simulink model "ADAC_AEBS_Test_B3_cs"  (Simulink 7.6)
settings: Solver=ode5  SolverMode=SingleTasking  StartTime=0.0  StopTime=inf  FixedStep=1/100  RelTol=1e-3
model workspace (MAT data in the model file):
  mbox_table : struct (value not decoded)
  model_closed = 0
  sim_status = 0
PreLoadFcn:
  | check_NUTS_defined;
  | 
  | assignin('base',['model_closed_' bdroot],false);addpath('../includes_AEBS');
InitFcn:
  | PreScanExperimentInitFcn(bdroot)
StopFcn:
  | PreScanExperimentStopFcn(bdroot)
undefined symbols (not defined in the file): DiscIntNeverNeededParam, x_ini_VRML, y_ini_VRML, z_ini_VRML
libraries: simulink x24, PreScanSimulinkLibrary x12, simulink_extras x7, PreScanUsefulBlocks x5, simulink_need_slupdate x1
(part 1 of 5)
CloseFcn:
  | evalin('base',['clear model_closed_' bdroot]);
settings Model: Creator=PRESCAN  LastModifiedBy=buildbot  BufferReuse=off
settings OptimizationCC: OptimizeBlockIOStorage=off  BufferReuse=off  ExpressionFolding=off  LocalBlockOutputs=off  InitFltsAndDblsToZero=on
settings DebuggingCC: SaveWithParameterizedLinksMsg=none  SignalResolutionControl=TryResolveAllWithWarning  SolverPrmCheckMsg=none  MultiTaskDSMMsg=warning  MultiTaskCondExecSysMsg=none
settings RTWCC: IncludeERTFirstTime=on
settings GRTTargetCC: TargetFcnLib=ansi_tfl_tmw.mat

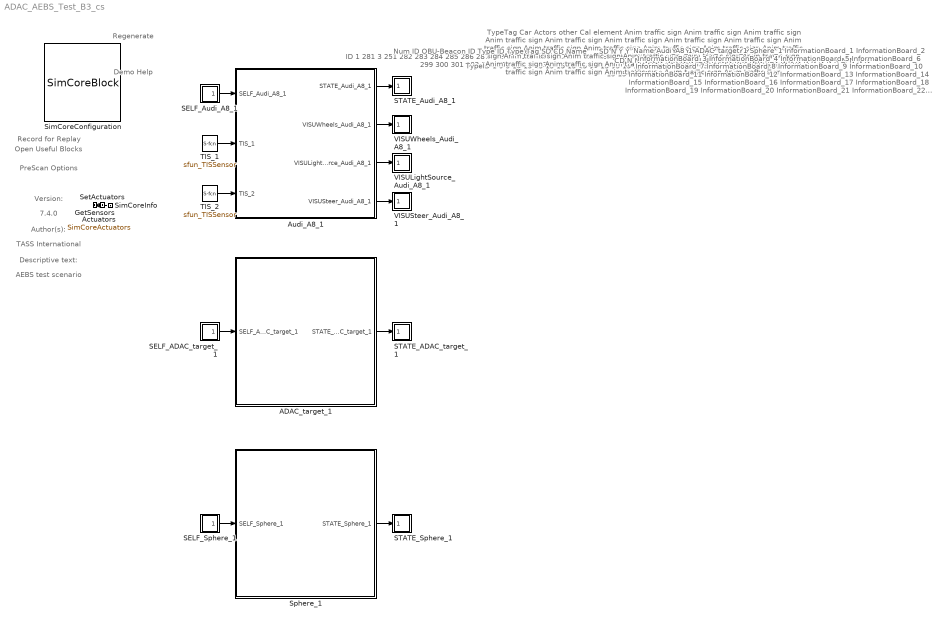
== system ADAC_AEBS_Test_B3_cs ==
  note: Demo Help
  note: Regenerate
  note: Record for Replay
  note: Open Useful Blocks
  note: PreScan Options
  note: Version:
  note: 7.4.0
  note: Author(s):
  note: TASS International
  note: Descriptive text:
  note: AEBS test scenario
  note: ID
      |
      | 1
      | 281
      | 3
      | 251
      | 282
      | 283
      | 284
      | 285
      | 286
      | 287
      | 288
      | 289
      | 290
      | 291
      | 292
      | 293
      | 294
      | 295
      | 296
      | 297
      | 298
      | 299
      | 300
      | 301
      | 302
      | 303
      | 304
      | 305
      | 306
      | 307
      | 308
      | 309
  note: OBU-Beacon ID
  note: TypeID
      |
      | 1
      | 9
      | 5
      | 15
      | 15
      | 15
      | 15
      | 15
      | 15
      | 15
      | 15
      | 15
      | 15
      | 15
      | 15
      | 15
      | 15
      | 15
      | 15
      | 15
      | 15
      | 15
      | 15
      | 15
      | 15
      | 15
      | 15
      | 15
      | 15
      | 15
      | 15
      | 15
  note: TypeTag
      |
      | Car
      | Actors other
      | Cal element
      | Anim traffic sign
      | Anim traffic sign
      | Anim traffic sign
      | Anim traffic sign
      | Anim traffic sign
      | Anim traffic sign
      | Anim traffic sign
      | Anim traffic sign
      | Anim traffic sign
      | Anim traffic sign
      | Anim traffic sign
      | Anim traffic sign
      | Anim traffic sign
      | Anim traffic sign
      | Anim traffic sign
      | Anim traffic sign
      | Anim traffic sign
      | Anim traffic sign
      | Anim traffic sign
      | Anim traffic sign
      | Anim traffic sign
      | Anim traffic sign
      | Anim traffic sign
      | Anim traffic sign
      | Anim traffic sign
      | Anim traffic sign
      | Anim traffic sign
      | Anim traffic sign
      | Anim traffic sign
  note: SD
      |
      | N
      | Y
      | Y
      | Y
      | Y
      | Y
      | Y
      | Y
      | Y
      | Y
      | Y
      | Y
      | Y
      | Y
      | Y
      | Y
      | Y
      | Y
      | Y
      | Y
      | Y
      | Y
      | Y
      | Y
      | Y
      | Y
      | Y
      | Y
      | Y
      | Y
      | Y
      | Y
  note: CD
      |
      | N
      | N
      | N
      | N
      | N
      | N
      | N
      | N
      | N
      | N
      | N
      | N
      | N
      | N
      | N
      | N
      | N
      | N
      | N
      | N
      | N
      | N
      | N
      | N
      | N
      | N
      | N
      | N
      | N
      | N
      | N
      | N
  note: Name
      |
      | Audi_A8_1
      | ADAC_target_1
      | Sphere_1
      | InformationBoard_1
      | InformationBoard_2
      | InformationBoard_3
      | InformationBoard_4
      | InformationBoard_5
      | InformationBoard_6
      | InformationBoard_7
      | InformationBoard_8
      | InformationBoard_9
      | InformationBoard_10
      | InformationBoard_11
      | InformationBoard_12
      | InformationBoard_13
      | InformationBoard_14
      | InformationBoard_15
      | InformationBoard_16
      | InformationBoard_17
      | InformationBoard_18
      | InformationBoard_19
      | InformationBoard_20
      | InformationBoard_21
      | InformationBoard_22
      | InformationBoard_23
      | InformationBoard_24
      | InformationBoard_25
      | InformationBoard_26
      | InformationBoard_27
      | InformationBoard_28
      | InformationBoard_29
  note: Num ID OBU-Beacon ID Type ID Type Tag SD CD Name
  ADAC_target_1 : Subsystem  Tag=WorldObjectSubSystem  InitFcn=UniqueId = '402';
      mask Display: image(imread('ADAC_target.jpg'));color('white');text(0,0,' ID=281\n')
  Actuators : DataStoreMemory  Tag=Actuators  DataStoreName=SimCoreActuators  InitialValue=zeros(273,1)
      settings: DeleteFcn=PreScanBlockDeleteFcn;
  Audi_A8_1 : Subsystem  Tag=WorldObjectSubSystem  InitFcn=UniqueId = '13';
      mask Display: image(imread('Audi_A8.jpg'));color('white');text(0,0,' ID=1\n')
  GetSensors : Subsystem  Tag=GetSensors  Priority=2  mask(PreScan Simulation Core Block){NrOfSensors=24, TimeStep=1/100}
      mask prompts: NrOfSensors "Number of sensor values"; TimeStep "Timestep [s]"
      mask help:
      | Please do not remove this block from the PreScan compilation sheet,
      | as it contains essential configuration parameters for a PreScan simulation.
      settings: DeleteFcn=PreScanBlockDeleteFcn;
  SELF_ADAC_target_1 : Subsystem  Tag=SELF  Priority=3  mask(PreScan Source Block: SELF){PortName=SELF_ADAC_target_1, PortIndex=8, PortWidth=8, TimeStep=1/100}
      mask prompts: PortName "Auto-Assigned: Port Name [-]"; PortIndex "Auto-Assigned: Port Index [-]"; PortWidth "Auto-Assigned: Port Dimensions"; TimeStep "Auto-Assigned: Upload Period [s]"
      mask help:
      | The SELF port shows (state) information of the actor itself. The outputs are position in the experiment's axis system and the GPS coordinates, and the object's absolute velocity and compass heading.
      |
      | For more information, please click Help.
      settings: DeleteFcn=PreScanBlockDeleteFcn;
      mask Help: eval('openHelp(462)')
      mask Display: image(imread('GPS.png'))
  SELF_Audi_A8_1 : Subsystem  Tag=SELF  Priority=3  mask(PreScan Source Block: SELF){PortName=SELF_Audi_A8_1, PortIndex=0, PortWidth=8, TimeStep=1/100}
      mask prompts: PortName "Auto-Assigned: Port Name [-]"; PortIndex "Auto-Assigned: Port Index [-]"; PortWidth "Auto-Assigned: Port Dimensions"; TimeStep "Auto-Assigned: Upload Period [s]"
      mask help:
      | The SELF port shows (state) information of the actor itself. The outputs are position in the experiment's axis system and the GPS coordinates, and the object's absolute velocity and compass heading.
      |
      | For more information, please click Help.
      settings: DeleteFcn=PreScanBlockDeleteFcn;
      mask Help: eval('openHelp(462)')
      mask Display: image(imread('GPS.png'))
  SELF_Sphere_1 : Subsystem  Tag=SELF  Priority=3  mask(PreScan Source Block: SELF){PortName=SELF_Sphere_1, PortIndex=16, PortWidth=8, TimeStep=1/100}
      mask prompts: PortName "Auto-Assigned: Port Name [-]"; PortIndex "Auto-Assigned: Port Index [-]"; PortWidth "Auto-Assigned: Port Dimensions"; TimeStep "Auto-Assigned: Upload Period [s]"
      mask help:
      | The SELF port shows (state) information of the actor itself. The outputs are position in the experiment's axis system and the GPS coordinates, and the object's absolute velocity and compass heading.
      |
      | For more information, please click Help.
      settings: DeleteFcn=PreScanBlockDeleteFcn;
      mask Help: eval('openHelp(462)')
      mask Display: image(imread('GPS.png'))
  STATE_ADAC_target_1 : Subsystem  Tag=State  Priority=0  mask(PreScan Sink Block: State){x0=128, y0=0, z0=0, Roll0=0, Pitch0=0, Yaw0=0, TimeStep=1/100}
      mask prompts: x0 "Ini x-position VEHICLE wrt GLOBAL axis system [m]"; y0 "Ini y-position VEHICLE wrt GLOBAL axis system [m]"; z0 "Ini z-position VEHICLE wrt GLOBAL axis system [m]"; Roll0 "Ini roll-angle BODY wrt VEHICLE axis system [deg]"; Pitch0 "Ini pitch-angle BODY wrt VEHICLE axis system [deg]"; Yaw0 "Ini yaw-angle VEHICLE wrt GLOBAL axis system [deg]"; TimeStep "Time Step [s]"
      mask help:
      | The Actor State contains a vector signal of size (9x1), containing the following signals:
      |
      | -  Position                  (x,y,z)                                     [m]
      | -  Velocity                  (vx,vy,vz)                               [m/s]
      | -  Angles                    (Roll, Pitch, Yaw)                   [rad]
      |
      | The Actor state is defined in the global axis system.
      | The state is superponed on the Initial position defined in the GUI.
      |
      | For more information, please click Help.
      settings: DeleteFcn=PreScanBlockDeleteFcn;
      mask Help: eval('openHelp(222)')
      mask Display: image(imread('State.png'))
  STATE_Audi_A8_1 : Subsystem  Tag=State  Priority=0  mask(PreScan Sink Block: State){x0=-2, y0=0, z0=0.550000011920929, Roll0=0, Pitch0=0, Yaw0=0, TimeStep=1/100}
      mask prompts: x0 "Ini x-position VEHICLE wrt GLOBAL axis system [m]"; y0 "Ini y-position VEHICLE wrt GLOBAL axis system [m]"; z0 "Ini z-position VEHICLE wrt GLOBAL axis system [m]"; Roll0 "Ini roll-angle BODY wrt VEHICLE axis system [deg]"; Pitch0 "Ini pitch-angle BODY wrt VEHICLE axis system [deg]"; Yaw0 "Ini yaw-angle VEHICLE wrt GLOBAL axis system [deg]"; TimeStep "Time Step [s]"
      mask help:
      | The Actor State contains a vector signal of size (9x1), containing the following signals:
      |
      | -  Position                  (x,y,z)                                     [m]
      | -  Velocity                  (vx,vy,vz)                               [m/s]
      | -  Angles                    (Roll, Pitch, Yaw)                   [rad]
      |
      | The Actor state is defined in the global axis system.
      | The state is superponed on the Initial position defined in the GUI.
      |
      | For more information, please click Help.
      settings: DeleteFcn=PreScanBlockDeleteFcn;
      mask Help: eval('openHelp(222)')
      mask Display: image(imread('State.png'))
  STATE_Sphere_1 : Subsystem  Tag=State  Priority=0  mask(PreScan Sink Block: State){x0=-2, y0=0, z0=0.550000011920929, Roll0=0, Pitch0=0, Yaw0=0, TimeStep=1/100}
      mask prompts: x0 "Ini x-position VEHICLE wrt GLOBAL axis system [m]"; y0 "Ini y-position VEHICLE wrt GLOBAL axis system [m]"; z0 "Ini z-position VEHICLE wrt GLOBAL axis system [m]"; Roll0 "Ini roll-angle BODY wrt VEHICLE axis system [deg]"; Pitch0 "Ini pitch-angle BODY wrt VEHICLE axis system [deg]"; Yaw0 "Ini yaw-angle VEHICLE wrt GLOBAL axis system [deg]"; TimeStep "Time Step [s]"
      mask help:
      | The Actor State contains a vector signal of size (9x1), containing the following signals:
      |
      | -  Position                  (x,y,z)                                     [m]
      | -  Velocity                  (vx,vy,vz)                               [m/s]
      | -  Angles                    (Roll, Pitch, Yaw)                   [rad]
      |
      | The Actor state is defined in the global axis system.
      | The state is superponed on the Initial position defined in the GUI.
      |
      | For more information, please click Help.
      settings: DeleteFcn=PreScanBlockDeleteFcn;
      mask Help: eval('openHelp(222)')
      mask Display: image(imread('State.png'))
  SetActuators : Subsystem  Tag=SetActuators  Priority=1  mask(PreScan Simulation Core Block){TimeStep=1/100, NrOfActuators=273}
      mask prompts: TimeStep "Timestep [s]"; NrOfActuators "Number of actuator values"
      mask help:
      | Please do not remove this block from the PreScan compilation sheet,
      | as it contains essential configuration parameters for a PreScan simulation.
      settings: DeleteFcn=PreScanBlockDeleteFcn;
  SimCoreConfiguration : M-S-Function  Tag=SimCoreConfiguration  Description=956F042E7F661D7092DC54456114AB9A9416500EBD947CDBFDED334F67B644E2  FunctionName=SimCoreBlock  Parameters=ExperimentXML PortsXML SimulationCore HostName CheckStart EnableLog RfR EnableGPUAccel ShowComputationTime  mask(PreScan Simulation Core Configurator){SimulationCore=NUTS, HostName=0, CheckStart=0, prescanversion='7.4.0', EnableLog=off, RfR=0, EnableGPUAccel=off, ShowComputationTime=off}
      mask prompts: SimulationCore "Simulation Core"; HostName "Simulation Host"; CheckStart "Show START Dialog"; prescanversion "PreScan Version"; EnableLog "Create TA Log"; RfR "Record for Replay"; EnableGPUAccel "Enable GPU Acceleration"; ShowComputationTime "Show ComputationTime Scope"
      mask help:
      | Please do not remove this block from the PreScan compilation sheet,
      | as it contains essential configuration parameter for a PreScan simulation.
      mask init:
      | model = bdroot;
      | ExperimentXML = [model(1:end-3) '.pex'];
      | PortsXML = [model '_ports.pcd'];
      settings: DeleteFcn=PreScanBlockDeleteFcn;  ModelCloseFcn=assignin('base',['model_closed_' bdroot],true);
      mask Help: eval('openHelp(812)')
      mask Display: image(imread('prescanlogo.ico'))
  SimCoreInfo : Subsystem  Tag=SimCoreInfo
  Sphere_1 : Subsystem  Tag=WorldObjectSubSystem  InitFcn=UniqueId = '409';
      mask Display: image(imread('Sphere.jpg'));color('white');text(0,0,' ID=3\n')
  TIS_1 : S-Function  Priority=3  LoadFcn=load('PrescanScannerSensorData.mat');load('PrescanScannerSensorMessage.mat')  FunctionName=sfun_TISSensor  Parameters=timestepMask maxInputMessages maxOutputMessages sensorID detectableObjects  EnableBusSupport=off  mask{timestepMask=1/25, maxInputMessages=0, maxOutputMessages=32, sensorID=14, detectableObjects=32}
      mask prompts: timestepMask "MATLAB timestep:"; maxInputMessages "Max input messages:"; maxOutputMessages "Max output messages:"; sensorID "Sensor ID:"; detectableObjects "Max detectable objects:"
      mask help: TIS Sensor I/O
      mask Display: image(imread('TIS.png'))
  TIS_2 : S-Function  Priority=3  LoadFcn=load('PrescanScannerSensorData.mat');load('PrescanScannerSensorMessage.mat')  FunctionName=sfun_TISSensor  Parameters=timestepMask maxInputMessages maxOutputMessages sensorID detectableObjects  EnableBusSupport=off  mask{timestepMask=1/25, maxInputMessages=0, maxOutputMessages=32, sensorID=15, detectableObjects=32}
      mask prompts: timestepMask "MATLAB timestep:"; maxInputMessages "Max input messages:"; maxOutputMessages "Max output messages:"; sensorID "Sensor ID:"; detectableObjects "Max detectable objects:"
      mask help: TIS Sensor I/O
      mask Display: image(imread('TIS.png'))
  VISULightSource_Audi_A8_1 : Subsystem  Tag=VisuLightSource  Priority=0
      settings: DeleteFcn=PreScanBlockDeleteFcn;
      mask Type: PreScan Sink Block: VisuLightSource
      mask Description:
      | The VisuLightSource block provides a way to animate Light Sources of the indicator, braking, fog and main lights of a vehicle.
      | 
      | For more information, please click Help.
      mask Help: eval('openHelp(223)')
      mask Display: image(imread('RearLight.png'))
  VISUSteer_Audi_A8_1 : Subsystem  Tag=VisuSteer  Priority=0
      settings: DeleteFcn=PreScanBlockDeleteFcn;
      mask Type: PreScan Sink Block: VisuSteer
      mask Description:
      | The VisuSteer block provides a way to adapt the orientation of the steering column and steering wheel of a vehicle.
      | 
      | For more information, please click Help.
      mask Help: eval('openHelp(223)')
      mask Display: image(imread('steeringwheel.png'))
  VISUWheels_Audi_A8_1 : Subsystem  Tag=VisuWheels  Priority=0
      settings: DeleteFcn=PreScanBlockDeleteFcn;
      mask Type: PreScan Sink Block: VisuWheels
      mask Description:
      | The VisuWheels block provides a way to animate the wheels of a vehicle, with steering, rotation (because of velocity) and z-displacement.
      | 
      | For more information, please click Help.
      mask Help: eval('openHelp(223)')
      mask Display: image(imread('wheel.png'))
  wires:
  Audi_A8_1/1(STATE_Audi_A8_1) -> STATE_Audi_A8_1/1(State)
  SELF_Audi_A8_1/1(U) -> Audi_A8_1/1(SELF_Audi_A8_1)
  TIS_1/1 -> Audi_A8_1/2(TIS_1)
  TIS_2/1 -> Audi_A8_1/3(TIS_2)
  Audi_A8_1/2(VISUWheels_Audi_A8_1) -> VISUWheels_Audi_A8_1/1(Wheels)
  Audi_A8_1/3(VISULightSource_Audi_A8_1) -> VISULightSource_Audi_A8_1/1(Lights)
  Audi_A8_1/4(VISUSteer_Audi_A8_1) -> VISUSteer_Audi_A8_1/1(Steer)
  ADAC_target_1/1(STATE_ADAC_target_1) -> STATE_ADAC_target_1/1(State)
  SELF_ADAC_target_1/1(U) -> ADAC_target_1/1(SELF_ADAC_target_1)
  Sphere_1/1(STATE_Sphere_1) -> STATE_Sphere_1/1(State)
  SELF_Sphere_1/1(U) -> Sphere_1/1(SELF_Sphere_1)
  SetActuators/1(dummy) -> GetSensors/1(dummy)

== system ADAC_AEBS_Test_B3_cs/ADAC_target_1 ==
  SELF_ADAC_target_1 : Inport  Tag=SELFInport
  SELF_Demux : Subsystem  Tag=DemuxSELF
      settings: DeleteFcn=PreScanBlockDeleteFcn;
      mask Type: PreScan Demux Block:
      mask Display:
      | port_label('output',1,'x [m]')
      | port_label('output',2,'y [m]')
      | port_label('output',3,'z [m]','texmode','on')
      | port_label('output',4,'Rotx [deg]','texmode','on')
      | port_label('output',5,'Roty [deg]','texmode','on')
      | port_label('output',6,'Rotz [deg]','texmode','on')
      | port_label('output',7,'GPS lat [deg]','texmode','on')
      | port_label('output',8,'GPS long [deg]','texmode','on')
      | port_label('output',9,'GPS alt [m]','texmode','on')
      | port_label('output',10,'Velocity [m/s]')
      | port_label('output',11,'Heading [deg]')
      | port_label('output',12,'Yaw rate [deg/s]')
  Terminator_{1..12} (12 alike) : Terminator
  Trajectories : Subsystem  Tag=Trajectories
      settings: DeleteFcn=PreScanBlockDeleteFcn;
      mask Type: PreScan Source Block: Trajectories
      mask Description:
      | The Trajectory block contains the trajectories defined in the PreScan Experiment Editor. The output of the trajectory block is the (vehicle) State.
      | 
      | For more information, please click Help.
      mask Help: eval('openHelp(312)')
      mask Display: image(imread('Trajectory.png'));
  STATE_ADAC_target_1 : Outport  Tag=StateOutport
  wires:
  SELF_ADAC_target_1/1 -> SELF_Demux/1(SELF)
  Trajectories/1(State) -> STATE_ADAC_target_1/1
  SELF_Demux/1(x [m]) -> Terminator_1/1
  SELF_Demux/2(y [m]) -> Terminator_2/1
  SELF_Demux/3(z [m]) -> Terminator_3/1
  SELF_Demux/4(rotx [deg]) -> Terminator_4/1
  SELF_Demux/5(roty [deg]) -> Terminator_5/1
  SELF_Demux/6(rotz [deg]) -> Terminator_6/1
  SELF_Demux/7(GPS lat [deg]) -> Terminator_7/1
  SELF_Demux/8(GPS long [deg]) -> Terminator_8/1
  SELF_Demux/9(GPS alt [m]) -> Terminator_9/1
  SELF_Demux/10(velocity [m/s]) -> Terminator_10/1
  SELF_Demux/11(heading [deg]) -> Terminator_11/1
  SELF_Demux/12(yaw rate [deg/s]) -> Terminator_12/1

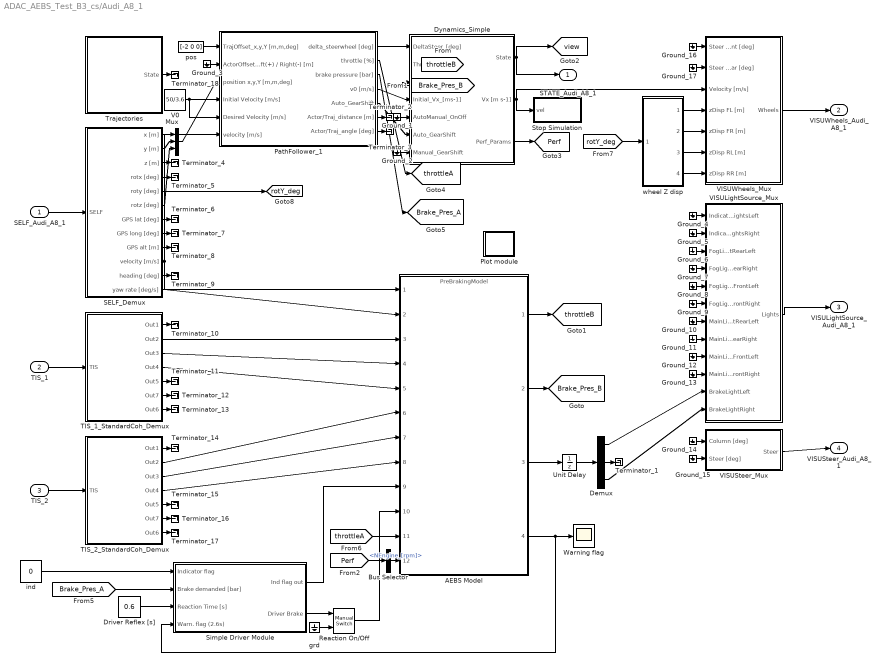
== system ADAC_AEBS_Test_B3_cs/Audi_A8_1 ==
  SELF_Audi_A8_1 : Inport  Tag=SELFInport
  TIS_1 : Inport  Tag=RadarInport  Port=2  OutDataTypeStr=Bus: PRESCAN_SCANNERSENSORMESSAGE
  TIS_2 : Inport  Tag=RadarInport  Port=3  OutDataTypeStr=Bus: PRESCAN_SCANNERSENSORMESSAGE
  AEBS Model : ModelReference  ModelNameDialog=PreBrakingModel  SimulationMode=Normal  ModelReferenceVersion=1.738  CopyOfModelName=PreBrakingModel
  Bus Selector : BusSelector  OutputSignals=NEngine_[rpm]
  Demux : Demux  Outputs=3
  Driver Reflex [s] : Constant  Value=0.6
  Dynamics_Simple : Subsystem  Tag=Simple_Vehicle_Dynamics  mask(PreScan Block: Simple Dynamics){Migrate=on, TimeStep=1/100, ComputationMode=Continuous_Time}
      mask prompts: Migrate "Migrate. During migration this block will be replaced by a newer one."; TimeStep "Auto assigned: Time Step [s]"; ComputationMode "Computation mode:"
      mask help:
      | The Simple Dynamics Model is selected in the GUI to simulate vehicle dynamics behavior.
      |
      | The Simple Dynamics Model is completely open to the user. The parameters of this model can be set in the Simple Dynamics dialog in the GUI.
      |
      | For more information, please click Help.
      mask init:
      | p = SimpleDyn_pars;
      settings: DeleteFcn=PreScanBlockDeleteFcn;
      mask Help: eval('openHelp(220)')
      mask Display:
      | image(imread('SimpleDyn.png'))
      | port_label('input', 1, '{\delta}_S_t_ _e_e_r [deg]','texmode','on')
      | port_label('input', 2, 'Throttle [%]')
      | port_label('input', 3, 'Brake Pres [bar]')
      | port_label('input', 4, 'V_0 [ms-1]','texmode','on')
      | port_label('input', 5, 'Auto=[0]/Manual=[1]')
      | port_label('input', 6, 'Auto_GearShift')
      | port_label('input', 7, 'Manual_GearShift')
      | port_label('output', 1, 'State')
      | port_label('output', 2, 'Vx [ms-1]')
      | port_label('output', 3, 'Perf Params')
  Ground_{1..17} (17 alike) : Ground
  Mux : Mux  Inputs=3
  PathFollower_1 : Subsystem  Tag=pathFollower  mask(PreScan Block: Path Follower){Migrate=on, FileName='Trajectory_2.mat', TunableSteeringGain=1, XShifting_wrt_COG=0}
      mask prompts: Migrate "Migrate. During migration this block will be replaced by a newer one."; FileName "Trajectory Name"; TunableSteeringGain "TunableSteeringGain [-]"; XShifting_wrt_COG "XShifting_wrt_COG [m]"
      mask help:
      | The Path Follower Model is selected in the GUI to simulate driver behavior.
      |
      | For more information, please click Help.
      mask init:
      | load(['trajectories/',eval(FileName)])
      | traject=trajectory';
      | 
      | Traj_x=traject(:,2);
      | Traj_y=traject(:,3);
      | Traj_z=traject(:,4);
      | Traj_vx=traject(:,8);
      | Traj_vy=traject(:,9);
      | Traj_vz=traject(:,10);
      mask Help: eval('openHelp(232)')
  Plot module : Subsystem  StopFcn=|
      | eml.extrinsic('plotyy','AEBS_EGOplot');
      | AEBS_EGOplot;
  Reaction On/Off : simulink/Signal Routing/Manual Switch  SystemSampleTime=-1  sw=0  action=0  varsize=off
  SELF_Demux : Subsystem  Tag=DemuxSELF
      settings: DeleteFcn=PreScanBlockDeleteFcn;
      mask Type: PreScan Demux Block:
      mask Display:
      | port_label('output',1,'x [m]')
      | port_label('output',2,'y [m]')
      | port_label('output',3,'z [m]','texmode','on')
      | port_label('output',4,'Rotx [deg]','texmode','on')
      | port_label('output',5,'Roty [deg]','texmode','on')
      | port_label('output',6,'Rotz [deg]','texmode','on')
      | port_label('output',7,'GPS lat [deg]','texmode','on')
      | port_label('output',8,'GPS long [deg]','texmode','on')
      | port_label('output',9,'GPS alt [m]','texmode','on')
      | port_label('output',10,'Velocity [m/s]')
      | port_label('output',11,'Heading [deg]')
      | port_label('output',12,'Yaw rate [deg/s]')
  Simple Driver Module : Subsystem
  Stop Simulation : Subsystem
  TIS_1_StandardCoh_Demux : Subsystem  TreatAsAtomicUnit=on  mask(PreScan Demux Block: TIS){MAXMESSAGES=32}
      mask prompts: MAXMESSAGES "Number of Objects"
      mask Help: eval('openHelp(441)')
      mask Display:
      | port_label('input',1,'TIS')
      | port_label('output',1,'Beam ID [-]')
      | port_label('output',2,'Range [m]')
      | port_label('output',3,'DopplerVelocity [m/s]')
      | port_label('output',4,'{\theta} [deg]','texmode','on')
      | port_label('output',5,'{\phi} [deg]','texmode','on')
      | port_label('output',6,'Target ID [-]','texmode','on')
      | port_label('output',7,'TIS Data','texmode','on')
  TIS_2_StandardCoh_Demux : Subsystem  TreatAsAtomicUnit=on  mask(PreScan Demux Block: TIS){MAXMESSAGES=32}
      mask prompts: MAXMESSAGES "Number of Objects"
      mask Help: eval('openHelp(441)')
      mask Display:
      | port_label('input',1,'TIS')
      | port_label('output',1,'Beam ID [-]')
      | port_label('output',2,'Range [m]')
      | port_label('output',3,'DopplerVelocity [m/s]')
      | port_label('output',4,'{\theta} [deg]','texmode','on')
      | port_label('output',5,'{\phi} [deg]','texmode','on')
      | port_label('output',6,'Target ID [-]','texmode','on')
      | port_label('output',7,'TIS Data','texmode','on')
  Terminator_{1..18} (18 alike) : Terminator
  Trajectories : Subsystem  Tag=Trajectories
      settings: DeleteFcn=PreScanBlockDeleteFcn;
      mask Type: PreScan Source Block: Trajectories
      mask Description:
      | The Trajectory block contains the trajectories defined in the PreScan Experiment Editor. The output of the trajectory block is the (vehicle) State.
      | 
      | For more information, please click Help.
      mask Help: eval('openHelp(312)')
      mask Display: image(imread('Trajectory.png'));
  Unit Delay : UnitDelay  SampleTime=-1
  V0 : Constant  Value=50/3.6
  VISULightSource_Mux : Subsystem  Tag=MuxLightSource
      settings: DeleteFcn=PreScanBlockDeleteFcn;
      mask Type: PreScan Mux Block:
  VISUSteer_Mux : Subsystem  Tag=MuxSteer
      settings: DeleteFcn=PreScanBlockDeleteFcn;
      mask Type: PreScan Mux Block:
  VISUWheels_Mux : Subsystem  Tag=MuxWheels  mask(PreScan Mux Block:){TimeStep=1/100}
      mask prompts: TimeStep "Auto Assigned: Time Step [s]"
      settings: DeleteFcn=PreScanBlockDeleteFcn;
  Warning flag : Scope
      settings: TimeRange=1.8  YMin=-1  YMax=1
  grd : Ground
  ind : Constant  Value=0
  pos : Constant  Tag=pos  Value=[-2 0 0]
  wheel Z disp : Subsystem  InitFcn=a = 1.17;  mask{a=1.17, b=1.77}
      mask prompts: a "Distance to the front wheel from cars center of gravity [m]"; b "Distance to the back wheel from cars center of gravity [m]"
      mask help: Simple Dynamics parameters
  STATE_Audi_A8_1 : Outport  Tag=StateOutport
  VISUWheels_Audi_A8_1 : Outport  Tag=VisuWheelsOutport  Port=2  SampleTime=1/100
  VISULightSource_Audi_A8_1 : Outport  Tag=VisuLightsOutport  Port=3  SampleTime=1/100
  VISUSteer_Audi_A8_1 : Outport  Tag=VisuSteerOutport  Port=4  SampleTime=1/100
  tag scope: Brake_Pres_A=global, Brake_Pres_B=global, Perf=global, rotY_deg=global, throttleA=global, throttleB=global, view=global
  wires:
  AEBS Model/2 -> [Brake_Pres_B]
  AEBS Model/4 -> Warning flag/1, Simple Driver Module/4(Warn. flag (2.6s))
  AEBS Model/1 -> [throttleB]
  [Brake_Pres_A] -> Simple Driver Module/2(Brake demanded [bar])
  Driver Reflex [s]/1 -> Simple Driver Module/3(Reaction Time [s])
  ind/1 -> Simple Driver Module/1(Indicator flag)
  Simple Driver Module/2(Driver Brake) -> Reaction On/Off/1
  grd/1 -> Reaction On/Off/2
  AEBS Model/3 -> Unit Delay/1
  Simple Driver Module/1(Ind flag out) -> AEBS Model/9
  Reaction On/Off/1 -> AEBS Model/10
  [throttleA] -> AEBS Model/11
  [rotY_deg] -> wheel Z disp/1(rotY [deg])
  Unit Delay/1 -> Demux/1
  [Perf] -> Bus Selector/1
  Bus Selector/1 -> AEBS Model/12  "<NEngine_[rpm]>"
  pos/1 -> PathFollower_1/1(TrajOffset_x,y,Y [m,m,deg])
  SELF_Audi_A8_1/1 -> SELF_Demux/1(SELF)
  VISUWheels_Mux/1(Wheels) -> VISUWheels_Audi_A8_1/1
  VISULightSource_Mux/1(Lights) -> VISULightSource_Audi_A8_1/1
  VISUSteer_Mux/1(Steer) -> VISUSteer_Audi_A8_1/1
  Dynamics_Simple/2(Vx [m s-1]) -> VISUWheels_Mux/3(Velocity [m/s]), Stop Simulation/1(vel)
  PathFollower_1/1(delta_steerwheel [deg]) -> Dynamics_Simple/1(DeltaSteer_[deg])
  PathFollower_1/2(throttle [%]) -> [throttleA]
  PathFollower_1/3(brake pressure [bar]) -> [Brake_Pres_A]
  PathFollower_1/4(v0 [m/s]) -> Dynamics_Simple/4(Initial_Vx_[ms-1])
  PathFollower_1/5(Auto_GearShift) -> Dynamics_Simple/6(Auto_GearShift)
  Dynamics_Simple/1(State) -> STATE_Audi_A8_1/1, [view]
  TIS_2_StandardCoh_Demux/2(Out2) -> AEBS Model/6
  TIS_1_StandardCoh_Demux/2(Out2) -> AEBS Model/3
  TIS_2_StandardCoh_Demux/3(Out3) -> AEBS Model/7
  TIS_1_StandardCoh_Demux/3(Out3) -> AEBS Model/4
  wheel Z disp/4(zDisp RR [m]) -> VISUWheels_Mux/7(zDisp RR [m])
  wheel Z disp/3(zDisp RL [m]) -> VISUWheels_Mux/6(zDisp RL [m])
  wheel Z disp/2(zDisp FR [m]) -> VISUWheels_Mux/5(zDisp FR [m])
  wheel Z disp/1(zDisp FL [m]) -> VISUWheels_Mux/4(zDisp FL [m])
  SELF_Demux/5(roty [deg]) -> [rotY_deg]
  Demux/3 -> VISULightSource_Mux/12(BrakeLightRight)
  Demux/1 -> VISULightSource_Mux/11(BrakeLightLeft)
  V0/1 -> PathFollower_1/4(Initial Velocity [m/s]), PathFollower_1/5(Desired Velocity [m/s])
  Mux/1 -> PathFollower_1/3(position x,y,Y [m,m,deg])
  SELF_Demux/6(rotz [deg]) -> Mux/3
  SELF_Demux/2(y [m]) -> Mux/2
  SELF_Demux/1(x [m]) -> Mux/1
  Dynamics_Simple/3(Perf_Params) -> [Perf]
  [throttleB] -> Dynamics_Simple/2(Throttle)
  [Brake_Pres_B] -> Dynamics_Simple/3(Brake)
  SELF_Demux/10(velocity [m/s]) -> PathFollower_1/6(velocity [m/s]), AEBS Model/1
  SELF_Demux/12(yaw rate [deg/s]) -> AEBS Model/2
  TIS_1_StandardCoh_Demux/4(Out4) -> AEBS Model/5
  TIS_2_StandardCoh_Demux/4(Out4) -> AEBS Model/8
  TIS_1/1 -> TIS_1_StandardCoh_Demux/1(TIS)
  TIS_2/1 -> TIS_2_StandardCoh_Demux/1(TIS)
  Demux/2 -> Terminator_1/1
  Ground_1/1 -> Dynamics_Simple/5(AutoManual_OnOff)
  Ground_2/1 -> Dynamics_Simple/7(Manual_GearShift)
  Ground_3/1 -> PathFollower_1/2(ActorOffset_Left(+) / Right(-) [m])
  PathFollower_1/6(Actor/Traj_distance [m]) -> Terminator_2/1
  PathFollower_1/7(Actor/Traj_angle [deg]) -> Terminator_3/1
  SELF_Demux/3(z [m]) -> Terminator_4/1
  SELF_Demux/4(rotx [deg]) -> Terminator_5/1
  SELF_Demux/7(GPS lat [deg]) -> Terminator_6/1
  SELF_Demux/8(GPS long [deg]) -> Terminator_7/1
  SELF_Demux/9(GPS alt [m]) -> Terminator_8/1
  SELF_Demux/11(heading [deg]) -> Terminator_9/1
  TIS_1_StandardCoh_Demux/1(Out1) -> Terminator_10/1
  TIS_1_StandardCoh_Demux/5(Out5) -> Terminator_11/1
  TIS_1_StandardCoh_Demux/6(Out7) -> Terminator_12/1
  TIS_1_StandardCoh_Demux/7(Out6) -> Terminator_13/1
  TIS_2_StandardCoh_Demux/1(Out1) -> Terminator_14/1
  TIS_2_StandardCoh_Demux/5(Out5) -> Terminator_15/1
  TIS_2_StandardCoh_Demux/6(Out7) -> Terminator_16/1
  TIS_2_StandardCoh_Demux/7(Out6) -> Terminator_17/1
  Trajectories/1(State) -> Terminator_18/1
  Ground_4/1 -> VISULightSource_Mux/1(IndicatorLightsLeft)
  Ground_5/1 -> VISULightSource_Mux/2(IndicatorLightsRight)
  Ground_6/1 -> VISULightSource_Mux/3(FogLightRearLeft)
  Ground_7/1 -> VISULightSource_Mux/4(FogLightRearRight)
  Ground_8/1 -> VISULightSource_Mux/5(FogLightFrontLeft)
  Ground_9/1 -> VISULightSource_Mux/6(FogLightFrontRight)
  Ground_10/1 -> VISULightSource_Mux/7(MainLightRearLeft)
  Ground_11/1 -> VISULightSource_Mux/8(MainLightRearRight)
  Ground_12/1 -> VISULightSource_Mux/9(MainLightFrontLeft)
  Ground_13/1 -> VISULightSource_Mux/10(MainLightFrontRight)
  Ground_14/1 -> VISUSteer_Mux/1(Column [deg])
  Ground_15/1 -> VISUSteer_Mux/2(Steer [deg])
  Ground_16/1 -> VISUWheels_Mux/1(Steer Angle Front [deg])
  Ground_17/1 -> VISUWheels_Mux/2(Steer Angle Rear [deg])

== system ADAC_AEBS_Test_B3_cs/GetSensors ==
  dummy : Inport
  GetSensors : M-S-Function  FunctionName=GetSensorsBlock  Parameters=TimeStep NrOfSensors
  tag scope: SimCoreSensors=global
  wires:
  GetSensors/1 -> [SimCoreSensors]
  dummy/1 -> GetSensors/1

== system ADAC_AEBS_Test_B3_cs/SELF_ADAC_target_1 ==
  Selector : Selector  IndexMode=Zero-based  IndexOptions=Starting index (dialog)  Indices=PortIndex  OutputSizes=PortWidth(1)
  U : Outport
  wires:
  Selector/1 -> U/1
  [SimCoreSensors] -> Selector/1

== system ADAC_AEBS_Test_B3_cs/SELF_Audi_A8_1 ==
  Selector : Selector  IndexMode=Zero-based  IndexOptions=Starting index (dialog)  Indices=PortIndex  OutputSizes=PortWidth(1)
  U : Outport
  wires:
  Selector/1 -> U/1
  [SimCoreSensors] -> Selector/1

== system ADAC_AEBS_Test_B3_cs/SELF_Sphere_1 ==
  Selector : Selector  IndexMode=Zero-based  IndexOptions=Starting index (dialog)  Indices=PortIndex  OutputSizes=PortWidth(1)
  U : Outport
  wires:
  Selector/1 -> U/1
  [SimCoreSensors] -> Selector/1

== system ADAC_AEBS_Test_B3_cs/STATE_ADAC_target_1 ==
  State : Inport  SampleTime=TimeStep
  Acceleration : Subsystem  mask(ToSensorWorld){PortName=Acceleration_ADAC_target_1, PortIndex=249, PortWidth=3, TimeStep=1/100}
      mask prompts: PortName "Port Name [-]"; PortIndex "Index [-]"; PortWidth "Port Dimensions [-]"; TimeStep "Upload Period [s]"
      mask help: Sends signal(s) from Simulink to the Sensor World
      mask Help:
      | Sends signal(s) from Simulink to the Sensor World.
      | 
      | - Port Name [-]: specifies the name of the output terminal of the Simulink block.
      | - Index [-]: specifies the start position in the output vector sent to the Sensor World
      | - Port dimensions [-]: specifies the width (number of scalars) of the output port
      | - Upload period [s]: specifies the upload period (in seconds) of the port.
      mask Display: port_label('input', 1, PortName)
  Demux : Demux  Outputs=5
  Position : Subsystem  mask(ToSensorWorld){PortName=Position_ADAC_target_1, PortIndex=243, PortWidth=3, TimeStep=1/100}
      mask prompts: PortName "Port Name [-]"; PortIndex "Index [-]"; PortWidth "Port Dimensions [-]"; TimeStep "Upload Period [s]"
      mask help: Sends signal(s) from Simulink to the Sensor World
      mask Help:
      | Sends signal(s) from Simulink to the Sensor World.
      | 
      | - Port Name [-]: specifies the name of the output terminal of the Simulink block.
      | - Index [-]: specifies the start position in the output vector sent to the Sensor World
      | - Port dimensions [-]: specifies the width (number of scalars) of the output port
      | - Upload period [s]: specifies the upload period (in seconds) of the port.
      mask Display: port_label('input', 1, PortName)
  RPY : Subsystem  mask(ToSensorWorld){PortName=RPY_ADAC_target_1, PortIndex=252, PortWidth=3, TimeStep=1/100}
      mask prompts: PortName "Port Name [-]"; PortIndex "Index [-]"; PortWidth "Port Dimensions [-]"; TimeStep "Upload Period [s]"
      mask help: Sends signal(s) from Simulink to the Sensor World
      mask Help:
      | Sends signal(s) from Simulink to the Sensor World.
      | 
      | - Port Name [-]: specifies the name of the output terminal of the Simulink block.
      | - Index [-]: specifies the start position in the output vector sent to the Sensor World
      | - Port dimensions [-]: specifies the width (number of scalars) of the output port
      | - Upload period [s]: specifies the upload period (in seconds) of the port.
      mask Display: port_label('input', 1, PortName)
  Velocity : Subsystem  mask(ToSensorWorld){PortName=Velocity_ADAC_target_1, PortIndex=246, PortWidth=3, TimeStep=1/100}
      mask prompts: PortName "Port Name [-]"; PortIndex "Index [-]"; PortWidth "Port Dimensions [-]"; TimeStep "Upload Period [s]"
      mask help: Sends signal(s) from Simulink to the Sensor World
      mask Help:
      | Sends signal(s) from Simulink to the Sensor World.
      | 
      | - Port Name [-]: specifies the name of the output terminal of the Simulink block.
      | - Index [-]: specifies the start position in the output vector sent to the Sensor World
      | - Port dimensions [-]: specifies the width (number of scalars) of the output port
      | - Upload period [s]: specifies the upload period (in seconds) of the port.
      mask Display: port_label('input', 1, PortName)
  iniBODYAngles wrtVEH [rad] : Constant  Value=[Roll0 Pitch0 0]  SampleTime=TimeStep
  iniVEHAngles wrtGLOB [rad] : Constant  Value=[0 0 Yaw0]  SampleTime=TimeStep
  iniVEHposition wrtGLOB [m] : Constant  Value=[x0 y0 z0]  SampleTime=TimeStep
  state2FullState : PreScanSimulinkLibrary/state2FullState  SystemSampleTime=-1
  velRPY : Subsystem  mask(ToSensorWorld){PortName=velRPY_ADAC_target_1, PortIndex=255, PortWidth=3, TimeStep=1/100}
      mask prompts: PortName "Port Name [-]"; PortIndex "Index [-]"; PortWidth "Port Dimensions [-]"; TimeStep "Upload Period [s]"
      mask help: Sends signal(s) from Simulink to the Sensor World
      mask Help:
      | Sends signal(s) from Simulink to the Sensor World.
      | 
      | - Port Name [-]: specifies the name of the output terminal of the Simulink block.
      | - Index [-]: specifies the start position in the output vector sent to the Sensor World
      | - Port dimensions [-]: specifies the width (number of scalars) of the output port
      | - Upload period [s]: specifies the upload period (in seconds) of the port.
      mask Display: port_label('input', 1, PortName)
  wires:
  Demux/5 -> velRPY/1(Y)
  Demux/4 -> RPY/1(Y)
  Demux/3 -> Acceleration/1(Y)
  Demux/2 -> Velocity/1(Y)
  Demux/1 -> Position/1(Y)
  State/1 -> state2FullState/1
  state2FullState/1 -> Demux/1
  iniVEHposition wrtGLOB [m]/1 -> state2FullState/2
  iniBODYAngles wrtVEH [rad]/1 -> state2FullState/3
  iniVEHAngles wrtGLOB [rad]/1 -> state2FullState/4

== system ADAC_AEBS_Test_B3_cs/STATE_Audi_A8_1 ==
  State : Inport  SampleTime=TimeStep
  Acceleration : Subsystem  mask(ToSensorWorld){PortName=Acceleration_Audi_A8_1, PortIndex=6, PortWidth=3, TimeStep=1/100}
      mask prompts: PortName "Port Name [-]"; PortIndex "Index [-]"; PortWidth "Port Dimensions [-]"; TimeStep "Upload Period [s]"
      mask help: Sends signal(s) from Simulink to the Sensor World
      mask Help:
      | Sends signal(s) from Simulink to the Sensor World.
      | 
      | - Port Name [-]: specifies the name of the output terminal of the Simulink block.
      | - Index [-]: specifies the start position in the output vector sent to the Sensor World
      | - Port dimensions [-]: specifies the width (number of scalars) of the output port
      | - Upload period [s]: specifies the upload period (in seconds) of the port.
      mask Display: port_label('input', 1, PortName)
  Demux : Demux  Outputs=5
  Position : Subsystem  mask(ToSensorWorld){PortName=Position_Audi_A8_1, PortIndex=0, PortWidth=3, TimeStep=1/100}
      mask prompts: PortName "Port Name [-]"; PortIndex "Index [-]"; PortWidth "Port Dimensions [-]"; TimeStep "Upload Period [s]"
      mask help: Sends signal(s) from Simulink to the Sensor World
      mask Help:
      | Sends signal(s) from Simulink to the Sensor World.
      | 
      | - Port Name [-]: specifies the name of the output terminal of the Simulink block.
      | - Index [-]: specifies the start position in the output vector sent to the Sensor World
      | - Port dimensions [-]: specifies the width (number of scalars) of the output port
      | - Upload period [s]: specifies the upload period (in seconds) of the port.
      mask Display: port_label('input', 1, PortName)
  RPY : Subsystem  mask(ToSensorWorld){PortName=RPY_Audi_A8_1, PortIndex=9, PortWidth=3, TimeStep=1/100}
      mask prompts: PortName "Port Name [-]"; PortIndex "Index [-]"; PortWidth "Port Dimensions [-]"; TimeStep "Upload Period [s]"
      mask help: Sends signal(s) from Simulink to the Sensor World
      mask Help:
      | Sends signal(s) from Simulink to the Sensor World.
      | 
      | - Port Name [-]: specifies the name of the output terminal of the Simulink block.
      | - Index [-]: specifies the start position in the output vector sent to the Sensor World
      | - Port dimensions [-]: specifies the width (number of scalars) of the output port
      | - Upload period [s]: specifies the upload period (in seconds) of the port.
      mask Display: port_label('input', 1, PortName)
  Velocity : Subsystem  mask(ToSensorWorld){PortName=Velocity_Audi_A8_1, PortIndex=3, PortWidth=3, TimeStep=1/100}
      mask prompts: PortName "Port Name [-]"; PortIndex "Index [-]"; PortWidth "Port Dimensions [-]"; TimeStep "Upload Period [s]"
      mask help: Sends signal(s) from Simulink to the Sensor World
      mask Help:
      | Sends signal(s) from Simulink to the Sensor World.
      | 
      | - Port Name [-]: specifies the name of the output terminal of the Simulink block.
      | - Index [-]: specifies the start position in the output vector sent to the Sensor World
      | - Port dimensions [-]: specifies the width (number of scalars) of the output port
      | - Upload period [s]: specifies the upload period (in seconds) of the port.
      mask Display: port_label('input', 1, PortName)
  iniBODYAngles wrtVEH [rad] : Constant  Value=[Roll0 Pitch0 0]  SampleTime=TimeStep
  iniVEHAngles wrtGLOB [rad] : Constant  Value=[0 0 Yaw0]  SampleTime=TimeStep
  iniVEHposition wrtGLOB [m] : Constant  Value=[x0 y0 z0]  SampleTime=TimeStep
  state2FullState : PreScanSimulinkLibrary/state2FullState  SystemSampleTime=-1
  velRPY : Subsystem  mask(ToSensorWorld){PortName=velRPY_Audi_A8_1, PortIndex=12, PortWidth=3, TimeStep=1/100}
      mask prompts: PortName "Port Name [-]"; PortIndex "Index [-]"; PortWidth "Port Dimensions [-]"; TimeStep "Upload Period [s]"
      mask help: Sends signal(s) from Simulink to the Sensor World
      mask Help:
      | Sends signal(s) from Simulink to the Sensor World.
      | 
      | - Port Name [-]: specifies the name of the output terminal of the Simulink block.
      | - Index [-]: specifies the start position in the output vector sent to the Sensor World
      | - Port dimensions [-]: specifies the width (number of scalars) of the output port
      | - Upload period [s]: specifies the upload period (in seconds) of the port.
      mask Display: port_label('input', 1, PortName)
  wires:
  Demux/5 -> velRPY/1(Y)
  Demux/4 -> RPY/1(Y)
  Demux/3 -> Acceleration/1(Y)
  Demux/2 -> Velocity/1(Y)
  Demux/1 -> Position/1(Y)
  State/1 -> state2FullState/1
  state2FullState/1 -> Demux/1
  iniVEHposition wrtGLOB [m]/1 -> state2FullState/2
  iniBODYAngles wrtVEH [rad]/1 -> state2FullState/3
  iniVEHAngles wrtGLOB [rad]/1 -> state2FullState/4

== system ADAC_AEBS_Test_B3_cs/STATE_Sphere_1 ==
  State : Inport  SampleTime=TimeStep
  Acceleration : Subsystem  mask(ToSensorWorld){PortName=Acceleration_Sphere_1, PortIndex=264, PortWidth=3, TimeStep=1/100}
      mask prompts: PortName "Port Name [-]"; PortIndex "Index [-]"; PortWidth "Port Dimensions [-]"; TimeStep "Upload Period [s]"
      mask help: Sends signal(s) from Simulink to the Sensor World
      mask Help:
      | Sends signal(s) from Simulink to the Sensor World.
      | 
      | - Port Name [-]: specifies the name of the output terminal of the Simulink block.
      | - Index [-]: specifies the start position in the output vector sent to the Sensor World
      | - Port dimensions [-]: specifies the width (number of scalars) of the output port
      | - Upload period [s]: specifies the upload period (in seconds) of the port.
      mask Display: port_label('input', 1, PortName)
  Demux : Demux  Outputs=5
  Position : Subsystem  mask(ToSensorWorld){PortName=Position_Sphere_1, PortIndex=258, PortWidth=3, TimeStep=1/100}
      mask prompts: PortName "Port Name [-]"; PortIndex "Index [-]"; PortWidth "Port Dimensions [-]"; TimeStep "Upload Period [s]"
      mask help: Sends signal(s) from Simulink to the Sensor World
      mask Help:
      | Sends signal(s) from Simulink to the Sensor World.
      | 
      | - Port Name [-]: specifies the name of the output terminal of the Simulink block.
      | - Index [-]: specifies the start position in the output vector sent to the Sensor World
      | - Port dimensions [-]: specifies the width (number of scalars) of the output port
      | - Upload period [s]: specifies the upload period (in seconds) of the port.
      mask Display: port_label('input', 1, PortName)
  RPY : Subsystem  mask(ToSensorWorld){PortName=RPY_Sphere_1, PortIndex=267, PortWidth=3, TimeStep=1/100}
      mask prompts: PortName "Port Name [-]"; PortIndex "Index [-]"; PortWidth "Port Dimensions [-]"; TimeStep "Upload Period [s]"
      mask help: Sends signal(s) from Simulink to the Sensor World
      mask Help:
      | Sends signal(s) from Simulink to the Sensor World.
      | 
      | - Port Name [-]: specifies the name of the output terminal of the Simulink block.
      | - Index [-]: specifies the start position in the output vector sent to the Sensor World
      | - Port dimensions [-]: specifies the width (number of scalars) of the output port
      | - Upload period [s]: specifies the upload period (in seconds) of the port.
      mask Display: port_label('input', 1, PortName)
  Velocity : Subsystem  mask(ToSensorWorld){PortName=Velocity_Sphere_1, PortIndex=261, PortWidth=3, TimeStep=1/100}
      mask prompts: PortName "Port Name [-]"; PortIndex "Index [-]"; PortWidth "Port Dimensions [-]"; TimeStep "Upload Period [s]"
      mask help: Sends signal(s) from Simulink to the Sensor World
      mask Help:
      | Sends signal(s) from Simulink to the Sensor World.
      | 
      | - Port Name [-]: specifies the name of the output terminal of the Simulink block.
      | - Index [-]: specifies the start position in the output vector sent to the Sensor World
      | - Port dimensions [-]: specifies the width (number of scalars) of the output port
      | - Upload period [s]: specifies the upload period (in seconds) of the port.
      mask Display: port_label('input', 1, PortName)
  iniBODYAngles wrtVEH [rad] : Constant  Value=[Roll0 Pitch0 0]  SampleTime=TimeStep
  iniVEHAngles wrtGLOB [rad] : Constant  Value=[0 0 Yaw0]  SampleTime=TimeStep
  iniVEHposition wrtGLOB [m] : Constant  Value=[x0 y0 z0]  SampleTime=TimeStep
  state2FullState : PreScanSimulinkLibrary/state2FullState  SystemSampleTime=-1
  velRPY : Subsystem  mask(ToSensorWorld){PortName=velRPY_Sphere_1, PortIndex=270, PortWidth=3, TimeStep=1/100}
      mask prompts: PortName "Port Name [-]"; PortIndex "Index [-]"; PortWidth "Port Dimensions [-]"; TimeStep "Upload Period [s]"
      mask help: Sends signal(s) from Simulink to the Sensor World
      mask Help:
      | Sends signal(s) from Simulink to the Sensor World.
      | 
      | - Port Name [-]: specifies the name of the output terminal of the Simulink block.
      | - Index [-]: specifies the start position in the output vector sent to the Sensor World
      | - Port dimensions [-]: specifies the width (number of scalars) of the output port
      | - Upload period [s]: specifies the upload period (in seconds) of the port.
      mask Display: port_label('input', 1, PortName)
  wires:
  Demux/5 -> velRPY/1(Y)
  Demux/4 -> RPY/1(Y)
  Demux/3 -> Acceleration/1(Y)
  Demux/2 -> Velocity/1(Y)
  Demux/1 -> Position/1(Y)
  State/1 -> state2FullState/1
  state2FullState/1 -> Demux/1
  iniVEHposition wrtGLOB [m]/1 -> state2FullState/2
  iniBODYAngles wrtVEH [rad]/1 -> state2FullState/3
  iniVEHAngles wrtGLOB [rad]/1 -> state2FullState/4

== system ADAC_AEBS_Test_B3_cs/SetActuators ==
  Bus Creator : BusCreator  Inputs=1
  Data Store Read : DataStoreRead  DataStoreName=SimCoreActuators  SampleTime=TimeStep
  SendActuators : M-S-Function  FunctionName=SendActuatorsBlock  Parameters=TimeStep NrOfActuators
  dummy : Outport
  tag scope: SimCoreInfo=global
  wires:
  Bus Creator/1 -> [SimCoreInfo]  "SimCore"
  SendActuators/2 -> Bus Creator/1  "ComputationTime[s]"
  SendActuators/1 -> dummy/1
  Data Store Read/1 -> SendActuators/1

== system ADAC_AEBS_Test_B3_cs/SimCoreInfo ==
  Bus Selector : BusSelector  OutputSignals=ComputationTime[s]
  Time : Scope
      settings: TimeRange=10  YMin=0  YMax=0.5  SaveName=ComputationTime
  wires:
  Bus Selector/1 -> Time/1  "<ComputationTime[s]>"
  [SimCoreInfo] -> Bus Selector/1

== system ADAC_AEBS_Test_B3_cs/Sphere_1 ==
  SELF_Sphere_1 : Inport  Tag=SELFInport
  Dynamics_Empty : Subsystem  Tag=Dynamics_Empty
      mask Display: port_label('output', 1, 'State');text(0,0,' Empty\n')
  Gain : Gain  Gain=[1 1 1 1 1 1 0 0 0]
  SELF_Demux : Subsystem  Tag=DemuxSELF
      settings: DeleteFcn=PreScanBlockDeleteFcn;
      mask Type: PreScan Demux Block:
      mask Display:
      | port_label('output',1,'x [m]')
      | port_label('output',2,'y [m]')
      | port_label('output',3,'z [m]','texmode','on')
      | port_label('output',4,'Rotx [deg]','texmode','on')
      | port_label('output',5,'Roty [deg]','texmode','on')
      | port_label('output',6,'Rotz [deg]','texmode','on')
      | port_label('output',7,'GPS lat [deg]','texmode','on')
      | port_label('output',8,'GPS long [deg]','texmode','on')
      | port_label('output',9,'GPS alt [m]','texmode','on')
      | port_label('output',10,'Velocity [m/s]')
      | port_label('output',11,'Heading [deg]')
      | port_label('output',12,'Yaw rate [deg/s]')
  Terminator_{1..13} (13 alike) : Terminator
  STATE_Sphere_1 : Outport  Tag=StateOutport
  wires:
  [view] -> Gain/1
  SELF_Sphere_1/1 -> SELF_Demux/1(SELF)
  Gain/1 -> STATE_Sphere_1/1
  Dynamics_Empty/1(State) -> Terminator_1/1
  SELF_Demux/1(x [m]) -> Terminator_2/1
  SELF_Demux/2(y [m]) -> Terminator_3/1
  SELF_Demux/3(z [m]) -> Terminator_4/1
  SELF_Demux/4(rotx [deg]) -> Terminator_5/1
  SELF_Demux/5(roty [deg]) -> Terminator_6/1
  SELF_Demux/6(rotz [deg]) -> Terminator_7/1
  SELF_Demux/7(GPS lat [deg]) -> Terminator_8/1
  SELF_Demux/8(GPS long [deg]) -> Terminator_9/1
  SELF_Demux/9(GPS alt [m]) -> Terminator_10/1
  SELF_Demux/10(velocity [m/s]) -> Terminator_11/1
  SELF_Demux/11(heading [deg]) -> Terminator_12/1
  SELF_Demux/12(yaw rate [deg/s]) -> Terminator_13/1
